simulink model "parte1"  (Simulink 8.1)
settings: Solver=ode113  StartTime=0.0  StopTime=5  FixedStep=0.05
values from neighbouring files (symbols this model uses):
  T = [0 0 0 0 0 0]    [parte1.m]
libraries: roblocks x1
settings Model: Creator=dello  LastModifiedBy=dello
settings DataIOCC: SignalLoggingSaveFormat=Dataset
settings OptimizationCC: ExpressionDepthLimit=128
settings DebuggingCC: FcnCallInpInsideContextMsg=EnableAllAsError
settings GRTTargetCC: CombineOutputUpdateFcns=on  GRTInterface=off

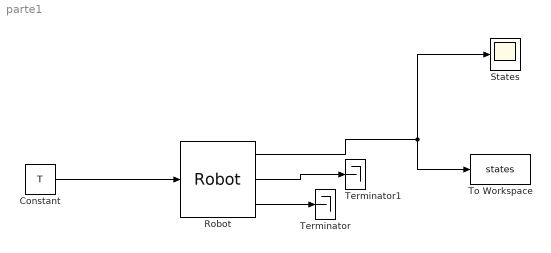
== system parte1 ==
  Constant : Constant  Value=T
  Robot : roblocks/Dynamics/Robot  robot=bot  q0=q0
  States : Scope
      settings: YMin=-4e-10  YMax=2.5e-11
  Terminator : Terminator
  Terminator1 : Terminator
  To Workspace : ToWorkspace  VariableName=states  SampleTime=-1  SaveFormat=Timeseries
  wires:
  Constant/1 -> Robot/1
  Robot/1 -> States/1, To Workspace/1
  Robot/3 -> Terminator/1
  Robot/2 -> Terminator1/1
